simulink model "double_pendulum_model"  (R2020a)
settings: Solver=FixedStepAuto  StartTime=0.0  StopTime=5  FixedStep=1e-4  RelTol=1e-3  AbsTol=1e-3  EnableMultiTasking=on
undefined symbols (not defined in the file): sigbuilder_block, X, Y, Z
libraries: sm_lib x13, nesl_utility x8, simulink_extras x6, fl_lib x3
settings Model: Creator=Albert  LastModifiedBy=Albert
settings SolverCC: AutoScaleAbsTol=off
settings DataIOCC: LimitDataPoints=on  MaxDataPoints=10000
settings OptimizationCC: LifeSpan=inf
settings DebuggingCC: AllowSymbolicDim=off  SFUnexpectedBacktrackingDiag=warning  SFNoUnconditionalDefaultTransitionDiag=warning  SFExecutionAtInitializationDiag=none  ArithmeticOperatorsInVariantConditions=warning
settings SFSimCC: SimUseLocalCustomCode=off  CustomCodeUndefinedFunction=UseInterfaceOnly
settings RTWCC: RTWUseLocalCustomCode=off
settings CodeAppCC: StateflowObjectComments=on
settings GRTTargetCC: TargetLangStandard=C89/C90 (ANSI)
settings ConfigComp: CovMetricSettings=dw  CovSaveCumulativeToWorkspaceVar=on  CovSaveSingleToWorkspaceVar=on  CovExternalEMLEnable=off  CovSFcnEnable=off
settings SimscapeCC: SimscapeLogType=all  SimscapeLogSimulationStatistics=on  SimscapeLogDataHistory=10000

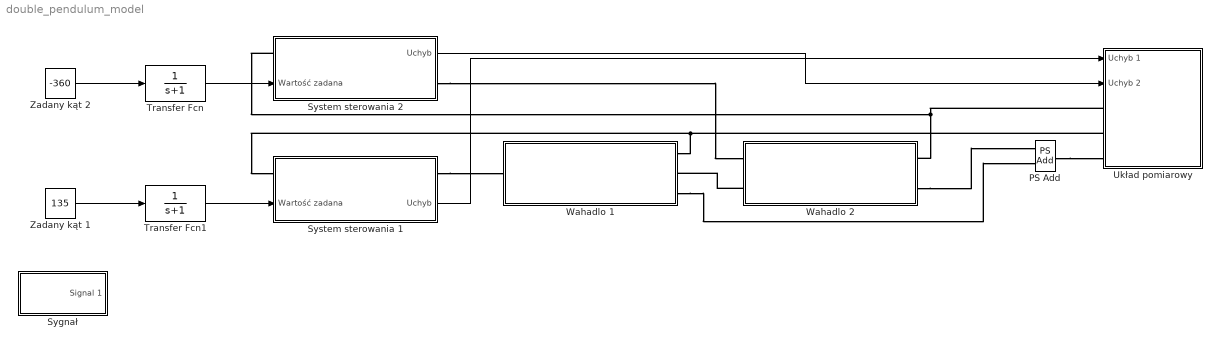
== system double_pendulum_model ==
  PS Add : fl_lib/Physical Signals/Functions/PS Add
  Sygnał : Subsystem  Tag=STV Subsys  LoadFcn=sigbuilder_block('load');  StartFcn=sigbuilder_block('start');  StopFcn=sigbuilder_block('stop');  ClipboardFcn=sigbuilder_block('clipboard');  mask(Sigbuilder block){tuvar=[0:10]}
      mask help: Simulink:masks:SigbuilderBlock_MD
      mask init:
      | if ~strcmp(get_param(bdroot(gcbh),'SimulationStatus'),'stopped') tuvar = sigbuilder_block('maskInit'); end
      settings: CopyFcn=sigbuilder_block('copy');  DeleteFcn=sigbuilder_block('delete');  ModelCloseFcn=sigbuilder_block('modelClose');  PreSaveFcn=sigbuilder_block('preSave');  PauseFcn=sigbuilder_block('pause');  ContinueFcn=sigbuilder_block('continue');  NameChangeFcn=sigbuilder_block('namechange');  OpenFcn=sigbuilder_block('open',[145.5 98.25 574.5 585.75 ]);  CloseFcn=sigbuilder_block('close');
      mask Display: plot(0, 0, 100, 100,[2, 2, 32, 32, 2], [68, 8, 8, 68, 68],[32, 2], [38, 38], [32, 19, 2],[53, 60, 44], [32, 17, 17, 2],[16, 16, 31, 31]);txt = getActiveGroup(gcbh);text(2, 100, txt,'verticalAlignment', 'top');
  System sterowania 1 : Subsystem
      settings: PortSchema="{\"entries\":[{\"content\":{\"sides\":[{\"content\":{\"connectorIds\":[\"LConn1\",\"In1\"]},\"type\":\"ConnectorPlacement.EquallySpacedRectSide\",\"uuid\":\"471d3fbd-ac29-446a-9427-316a60a908e6\"},{\"content\":{\"connectorIds\":[\"RConn1\",\"Out1\"],\"side\":\"RIGHT\"},\"type\":\"ConnectorPlacement.EquallySpacedRectSide\",\"uuid\":\"4c631136-7496-42ce-9ab5-63d38de6795d\"},{\"content\":{\"connectorIds\":[],\"side\":\"TOP\"},\"type\":\"ConnectorPlacement.EquallySpacedRectSide\",\"uuid\":\"d7f460c4-eb30-472b-8229-d5705620fcfc\"}]},\"type\":\"ConnectorPlacement.EquallySpacedConnector\",\"uuid\":\"0e46a79e-6a4e-432a-b324-1adcc0c34b7a\"}],\"packageUris\":[\"http://schema.mathworks.com/mf0/Connector/R2020b\"],\"version\":\"1.0\"}"
  System sterowania 2 : Subsystem
      settings: PortSchema="{\"entries\":[{\"content\":{\"sides\":[{\"content\":{\"connectorIds\":[\"LConn1\",\"In1\"]},\"type\":\"ConnectorPlacement.EquallySpacedRectSide\",\"uuid\":\"471d3fbd-ac29-446a-9427-316a60a908e6\"},{\"content\":{\"connectorIds\":[\"Out1\",\"RConn1\"],\"side\":\"RIGHT\"},\"type\":\"ConnectorPlacement.EquallySpacedRectSide\",\"uuid\":\"4c631136-7496-42ce-9ab5-63d38de6795d\"},{\"content\":{\"connectorIds\":[],\"side\":\"TOP\"},\"type\":\"ConnectorPlacement.EquallySpacedRectSide\",\"uuid\":\"d7f460c4-eb30-472b-8229-d5705620fcfc\"}]},\"type\":\"ConnectorPlacement.EquallySpacedConnector\",\"uuid\":\"0e46a79e-6a4e-432a-b324-1adcc0c34b7a\"}],\"packageUris\":[\"http://schema.mathworks.com/mf0/Connector/R2020b\"],\"version\":\"1.0\"}"
  Transfer Fcn : TransferFcn  Denominator=[1 1]
  Transfer Fcn1 : TransferFcn  Denominator=[1 1]
  Układ pomiarowy : Subsystem
  Wahadlo 1 : Subsystem
  Wahadlo 2 : Subsystem
  Zadany kąt 1 : Constant  Value=135
  Zadany kąt 2 : Constant  Value=-360
  wires:
  System sterowania 2/1(Uchyb) -> Układ pomiarowy/2(Uchyb 2)
  System sterowania 1/1(Uchyb) -> Układ pomiarowy/1(Uchyb 1)
  Zadany kąt 1/1 -> Transfer Fcn1/1
  Zadany kąt 2/1 -> Transfer Fcn/1
  Transfer Fcn/1 -> System sterowania 2/1(Wartość zadana)
  Transfer Fcn1/1 -> System sterowania 1/1(Wartość zadana)
  connections:
  Wahadlo 1/RConn1 -- System sterowania 1/LConn1 -- Układ pomiarowy/LConn2
  System sterowania 1/RConn1 -- Wahadlo 1/LConn1
  Wahadlo 2/LConn2 -- Wahadlo 1/RConn2
  System sterowania 2/LConn1 -- Układ pomiarowy/LConn1 -- Wahadlo 2/RConn1
  PS Add/RConn1 -- Układ pomiarowy/LConn3
  Wahadlo 1/RConn3 -- PS Add/LConn2
  Wahadlo 2/RConn2 -- PS Add/LConn1
  System sterowania 2/RConn1 -- Wahadlo 2/LConn1

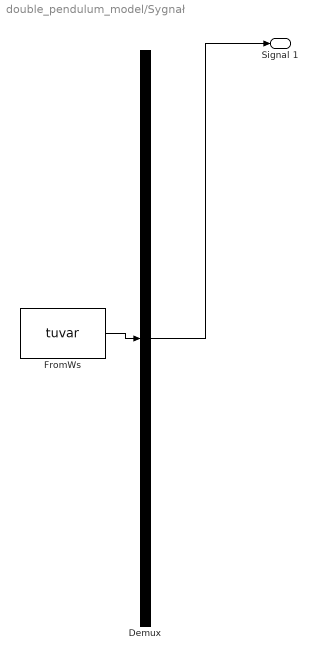
== system double_pendulum_model/Sygnał ==
  Demux : Demux  Tag=STV Demux  Outputs=1
      settings: DisplayOption=none
  FromWs : FromWorkspace  Tag=STV FromWs  VariableName=tuvar
      SigBuilderData=|
      | common.afterFinalStr = 'Extrapolate'
      | common.sampleTime = 0
      | dataSet.timeRange = [0 100]
      | dataSet.name = 'Group 1'
      | sbobj.Groups.Name = 'Group 1'
      | sbobj.Groups.Signals.Name = 'Signal 1'
      | sbobj.Groups.Signals.XData = [0 5 20 30 100]
      | sbobj.Groups.Signals.YData = [0 90 90 0 0]
      | sbobj.Groups.TimeRange = [0 100]
  Signal 1 : Outport  Tag=STV Outport  VectorParamsAs1DForOutWhenUnconnected=off
  wires:
  FromWs/1 -> Demux/1
  Demux/1 -> Signal 1/1

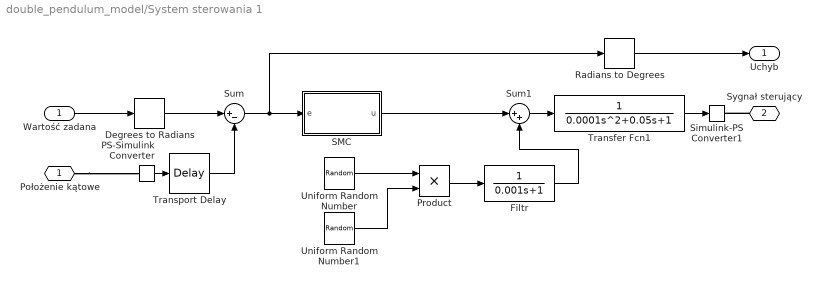
== system double_pendulum_model/System sterowania 1 ==
  Wartość zadana : Inport
  Degrees to Radians : simulink_extras/Transformations/Degrees to Radians
  Filtr : TransferFcn  Denominator=[0.001 1]
  PS-Simulink Converter : nesl_utility/PS-Simulink Converter  PhysicalDomain=network_engine_domain  SubClassName=ps_output  LeftPortType=input  RightPortType=output  PseudoPeriodic=off  Frequencies=[]  Unit=inherit  AffineConversion=off
      settings: SourceProductBaseCode=PW,SS
  Product : Product
  Radians to Degrees : simulink_extras/Transformations/Radians to Degrees
  SMC : Subsystem
  Simulink-PS Converter1 : nesl_utility/Simulink-PS Converter  PhysicalDomain=network_engine_domain  SubClassName=ps_input  LeftPortType=input  RightPortType=output  PseudoPeriodic=off  Frequencies=[]  NoiseDistribution=none  NoiseParameters=[]  Unit=1  AffineConversion=off  FilteringAndDerivatives=provide  SimscapeFilterOrder=1  InputFilterTimeConstant=0.001  UdotUserProvided=0
      settings: SourceProductBaseCode=PW,SS
  Sum : Sum  Inputs=|+-
  Sum1 : Sum  Inputs=|++
  Transfer Fcn1 : TransferFcn  Denominator=[0.0001 0.05 1]
  Transport Delay : TransportDelay  DelayTime=0.0001
  Uniform Random Number : UniformRandomNumber  Minimum=-0.05  Maximum=0.05
  Uniform Random Number1 : UniformRandomNumber  Minimum=-0.1  Maximum=0.1
  Położenie kątowe : PMIOPort  Side=Left
  Sygnał sterujący : PMIOPort  Port=2  Side=Right
  Uchyb : Outport
  wires:
  Degrees to Radians/1 -> Sum/1
  Wartość zadana/1 -> Degrees to Radians/1
  Sum/1 -> Radians to Degrees/1, SMC/1(e)
  PS-Simulink Converter/1 -> Transport Delay/1
  Transport Delay/1 -> Sum/2
  Uniform Random Number1/1 -> Product/2
  SMC/1(u) -> Sum1/1
  Uniform Random Number/1 -> Product/1
  Sum1/1 -> Transfer Fcn1/1
  Transfer Fcn1/1 -> Simulink-PS Converter1/1
  Product/1 -> Filtr/1
  Filtr/1 -> Sum1/2
  Radians to Degrees/1 -> Uchyb/1
  connections:
  Położenie kątowe/RConn1 -- PS-Simulink Converter/LConn1
  Sygnał sterujący/RConn1 -- Simulink-PS Converter1/RConn1

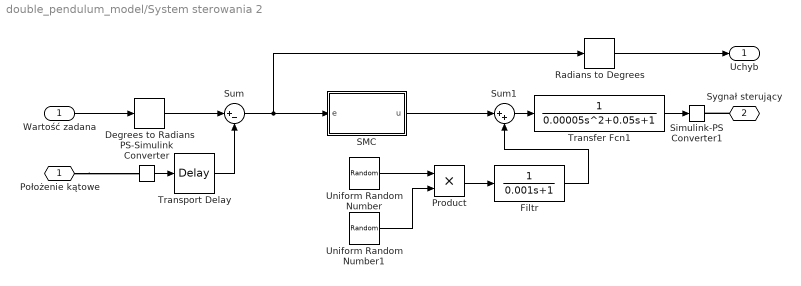
== system double_pendulum_model/System sterowania 2 ==
  Wartość zadana : Inport
  Degrees to Radians : simulink_extras/Transformations/Degrees to Radians
  Filtr : TransferFcn  Denominator=[0.001 1]
  PS-Simulink Converter : nesl_utility/PS-Simulink Converter  PhysicalDomain=network_engine_domain  SubClassName=ps_output  LeftPortType=input  RightPortType=output  PseudoPeriodic=off  Frequencies=[]  Unit=inherit  AffineConversion=off
      settings: SourceProductBaseCode=PW,SS
  Product : Product
  Radians to Degrees : simulink_extras/Transformations/Radians to Degrees
  SMC : Subsystem
  Simulink-PS Converter1 : nesl_utility/Simulink-PS Converter  PhysicalDomain=network_engine_domain  SubClassName=ps_input  LeftPortType=input  RightPortType=output  PseudoPeriodic=off  Frequencies=[]  NoiseDistribution=none  NoiseParameters=[]  Unit=1  AffineConversion=off  FilteringAndDerivatives=provide  SimscapeFilterOrder=1  InputFilterTimeConstant=0.001  UdotUserProvided=0
      settings: SourceProductBaseCode=PW,SS
  Sum : Sum  Inputs=|+-
  Sum1 : Sum  Inputs=|++
  Transfer Fcn1 : TransferFcn  Denominator=[0.00005 0.05 1]
  Transport Delay : TransportDelay  DelayTime=0.0001
  Uniform Random Number : UniformRandomNumber  Minimum=-0.05  Maximum=0.05
  Uniform Random Number1 : UniformRandomNumber  Minimum=-0.1  Maximum=0.1
  Położenie kątowe : PMIOPort  Side=Left
  Sygnał sterujący : PMIOPort  Port=2  Side=Right
  Uchyb : Outport
  wires:
  Sum/1 -> Radians to Degrees/1, SMC/1(e)
  Wartość zadana/1 -> Degrees to Radians/1
  Degrees to Radians/1 -> Sum/1
  PS-Simulink Converter/1 -> Transport Delay/1
  Transport Delay/1 -> Sum/2
  SMC/1(u) -> Sum1/1
  Uniform Random Number/1 -> Product/1
  Uniform Random Number1/1 -> Product/2
  Transfer Fcn1/1 -> Simulink-PS Converter1/1
  Sum1/1 -> Transfer Fcn1/1
  Product/1 -> Filtr/1
  Filtr/1 -> Sum1/2
  Radians to Degrees/1 -> Uchyb/1
  connections:
  Położenie kątowe/RConn1 -- PS-Simulink Converter/LConn1
  Sygnał sterujący/RConn1 -- Simulink-PS Converter1/RConn1

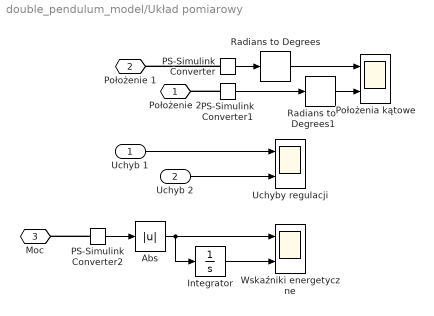
== system double_pendulum_model/Układ pomiarowy ==
  Uchyb 1 : Inport
  Uchyb 2 : Inport  Port=2
  Abs : Abs
  Integrator : Integrator
  PS-Simulink Converter : nesl_utility/PS-Simulink Converter  PhysicalDomain=network_engine_domain  SubClassName=ps_output  LeftPortType=input  RightPortType=output  PseudoPeriodic=off  Frequencies=[]  Unit=inherit  AffineConversion=off
      settings: SourceProductBaseCode=PW,SS
  PS-Simulink Converter1 : nesl_utility/PS-Simulink Converter  PhysicalDomain=network_engine_domain  SubClassName=ps_output  LeftPortType=input  RightPortType=output  PseudoPeriodic=off  Frequencies=[]  Unit=inherit  AffineConversion=off
      settings: SourceProductBaseCode=PW,SS
  PS-Simulink Converter2 : nesl_utility/PS-Simulink Converter  PhysicalDomain=network_engine_domain  SubClassName=ps_output  LeftPortType=input  RightPortType=output  PseudoPeriodic=off  Frequencies=[]  Unit=inherit  AffineConversion=off
      settings: SourceProductBaseCode=PW,SS
  Położenia kątowe : Scope  NumInputPorts=2
  Radians to Degrees : simulink_extras/Transformations/Radians to Degrees
  Radians to Degrees1 : simulink_extras/Transformations/Radians to Degrees
  Uchyby regulacji : Scope  NumInputPorts=2
  Wskaźniki energetyczne : Scope  NumInputPorts=2
  Położenie 2 : PMIOPort  Side=Left
  Położenie 1 : PMIOPort  Port=2  Side=Left
  Moc : PMIOPort  Port=3  Side=Left
  wires:
  Uchyb 2/1 -> Uchyby regulacji/2
  Uchyb 1/1 -> Uchyby regulacji/1
  Integrator/1 -> Wskaźniki energetyczne/2
  PS-Simulink Converter/1 -> Radians to Degrees/1
  Radians to Degrees/1 -> Położenia kątowe/1
  Radians to Degrees1/1 -> Położenia kątowe/2
  PS-Simulink Converter1/1 -> Radians to Degrees1/1
  PS-Simulink Converter2/1 -> Abs/1
  Abs/1 -> Wskaźniki energetyczne/1, Integrator/1
  connections:
  PS-Simulink Converter1/LConn1 -- Położenie 2/RConn1
  PS-Simulink Converter/LConn1 -- Położenie 1/RConn1
  PS-Simulink Converter2/LConn1 -- Moc/RConn1

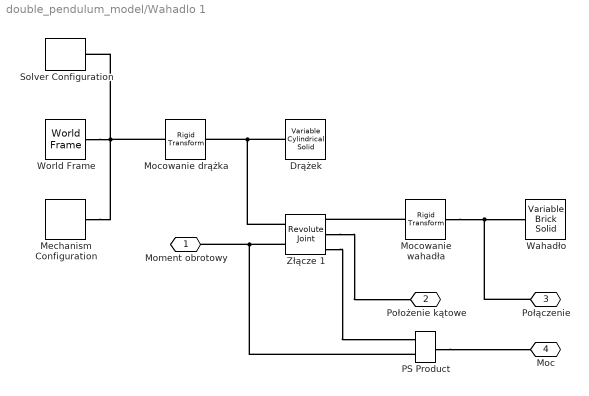
== system double_pendulum_model/Wahadlo 1 ==
  Drążek : sm_lib/Body Elements/Variable Mass/Variable Cylindrical Solid  LengthType=Constant  Length=50  LengthUnits=cm  RadiusType=Constant  Radius=30  RadiusUnits=mm  MassType=CalculateFromGeometry  InitialMassType=Specified  InitialMass=1  InitialMassUnits=kg  Density=1000  DensityUnits=kg/m^3  SenseRadius=off  SenseLength=off  SenseMass=off  SenseCenterOfMass=off  SenseInertiaMatrix=off  GraphicType=FromGeometry  MarkerShape=Sphere  MarkerSize=10  GraphicVisPropType=SimpleVisualProperties  GraphicDiffuseColor=[1.0 1.0 1.0]  GraphicSpecularColor=[0.5 0.5 0.5 1.0]  GraphicAmbientColor=[0.15 0.15 0.15 1.0]  GraphicEmissiveColor=[0.0 0.0 0.0 1.0]  GraphicShininess=75  GraphicOpacity=1.0
      settings: SourceProductBaseCode=MS
  Mechanism Configuration : sm_lib/Utilities/Mechanism Configuration  UniformGravity=Constant  GravityVector=[0 0 -9.80665]  GravityVectorUnits=m/s^2  GravityUnits=m/s^2  LinearizationDelta=0.001  JointModeTransitionNonlinearIterations=2
  Mocowanie drążka : sm_lib/Frames and Transforms/Rigid Transform  TranslationMethod=None  TranslationStandardOffset=0  TranslationLengthUnit=m  TranslationStandardAxis=+Z  TranslationCartesianOffset=[0 0 0]  TranslationROffset=0  TranslationROffsetUnits=m  TranslationZOffset=0  TranslationZOffsetUnits=m  TranslationThetaOffset=0  TranslationThetaOffsetUnits=deg  RotationMethod=RotationSequence  RotationAngleUnits=deg  RotationStandardAxis=+Z  RotationAngle=0.0  RotationArbitraryAxis=[0 0 1]  FollAlignAxisA=+X  BaseAlignAxisA=+Y  FollAlignAxisB=+Y  BaseAlignAxisB=+Z  RotationSequenceAxes=FollowerAxes  RotationSequence=YXY  RotationSequenceAngles=[0 90 0]  RotationSequenceAnglesUnits=deg  RotationMatrix=[1 0 0; 0 1 0; 0 0 1]
  Mocowanie wahadła : sm_lib/Frames and Transforms/Rigid Transform  TranslationMethod=Cartesian  TranslationStandardOffset=0  TranslationLengthUnit=cm  TranslationStandardAxis=+Z  TranslationCartesianOffset=[0 -14 25]  TranslationROffset=0  TranslationROffsetUnits=m  TranslationZOffset=0  TranslationZOffsetUnits=m  TranslationThetaOffset=0  TranslationThetaOffsetUnits=deg  RotationMethod=RotationSequence  RotationAngleUnits=deg  RotationStandardAxis=+Z  RotationAngle=0.0  RotationArbitraryAxis=[0 0 1]  FollAlignAxisA=+X  BaseAlignAxisA=+Y  FollAlignAxisB=+Y  BaseAlignAxisB=+Z  RotationSequenceAxes=FollowerAxes  RotationSequence=XYZ  RotationSequenceAngles=[0 0 90]  RotationSequenceAnglesUnits=deg  RotationMatrix=[1 0 0; 0 1 0; 0 0 1]
  PS Product : fl_lib/Physical Signals/Functions/PS Product
  Solver Configuration : nesl_utility/Solver Configuration  PhysicalDomain=network_engine_domain  SubClassName=solver  LeftPortType=input  RightPortType=generic  Tones=[]  Harmonics=[]  SimulateNoise=off  Profile=off  UseLocalSampling=off  EnableSwitchedLinearOptims=on  FrequencyDomain=off  UseCCode=off  RelTol=0.001  AbsTol=1e-06  MinStep=1e-09  ToWorkspace=off  RevertToSquareIcSolve=off  NumHomotopyIterations=100  PhasorMode=off  PhasorModeNumHarmonics=1  DoDC=off  ResidualTolerance=1e-09  UseLocalSolver=off  LocalSolverChoice=NE_BACKWARD_EULER_ADVANCER  LocalSolverSampleTime=0.001  DoFixedCost=off  MaxNonlinIter=3  MaxModeIter=2  ComputeImpulses=off  ImpulseIterations=2  LinearAlgebra=Sparse  EquationFormulation=NE_TIME_EF  DelaysMemoryBudget=1024  AutomaticFiltering=on  FilteringTimeConstant=0.001  PartitionStorageMethod=AS_NEEDED  PartitionMemoryBudget=1024  PartitionMethod=FAST
      settings: SourceProductBaseCode=PW,SS
  Wahadło : sm_lib/Body Elements/Variable Mass/Variable Brick Solid  XLengthType=Constant  XLength=30  XLengthUnits=cm  YLengthType=Constant  YLength=5  YLengthUnits=cm  ZLengthType=Constant  ZLength=20  ZLengthUnits=mm  MassType=CalculateFromGeometry  InitialMassType=Specified  InitialMass=1  InitialMassUnits=kg  Density=5000  DensityUnits=kg/m^3  SenseXLength=off  SenseYLength=off  SenseZLength=off  SenseMass=off  SenseCenterOfMass=off  SenseInertiaMatrix=off  GraphicType=FromGeometry  MarkerShape=Sphere  MarkerSize=10  GraphicVisPropType=SimpleVisualProperties  GraphicDiffuseColor=[1.0 0.0 0.0]  GraphicSpecularColor=[0.5 0.5 0.5 1.0]  GraphicAmbientColor=[0.15 0.15 0.15 1.0]  GraphicEmissiveColor=[0.0 0.0 0.0 1.0]  GraphicShininess=75  GraphicOpacity=0.5
      settings: SourceProductBaseCode=MS
  World Frame : sm_lib/Frames and Transforms/World Frame
  Złącze 1 : sm_lib/Joints/Revolute Joint  JointMode=Normal  SenseConstraintForce=off  SenseConstraintForceX=off  SenseConstraintForceY=off  SenseConstraintForceZ=off  SenseConstraintTorque=off  SenseConstraintTorqueX=off  SenseConstraintTorqueY=off  SenseConstraintTorqueZ=off  SenseTotalForce=off  SenseTotalForceX=off  SenseTotalForceY=off  SenseTotalForceZ=off  SenseTotalTorque=off  SenseTotalTorqueX=off  SenseTotalTorqueY=off  SenseTotalTorqueZ=off  CompositeWrenchDir=FollowerOnBase  CompositeWrenchFrame=BaseFrame  EquilibriumPosition=0  EquilibriumPositionUnits=deg  SpringStiffness=0  SpringStiffnessUnits=N*m/deg  DampingCoefficient=0.001  DampingCoefficientUnits=N*m/(deg/s)  TorqueActuationMode=InputTorque  MotionActuationMode=ComputedMotion  SensePosition=on  SenseVelocity=on  SenseAcceleration=off  SenseTorqueForce=off  SenseLowerLimitTorqueForce=off  SenseUpperLimitTorqueForce=off  LowerLimitSpecify=off  LowerLimitBound=-90  LowerLimitBoundUnits=deg  LowerLimitStiffness=1e4  LowerLimitStiffnessUnits=N*m/deg  LowerLimitDamping=10  LowerLimitDampingUnits=N*m/(deg/s)  LowerLimitTransitionRegionWidth=0.1  LowerLimitTransitionRegionWidthUnits=deg  UpperLimitSpecify=off  UpperLimitBound=90  UpperLimitBoundUnits=deg  UpperLimitStiffness=1e4  UpperLimitStiffnessUnits=N*m/deg  UpperLimitDamping=10  UpperLimitDampingUnits=N*m/(deg/s)  UpperLimitTransitionRegionWidth=0.1  UpperLimitTransitionRegionWidthUnits=deg  PositionTargetSpecify=off  PositionTargetPriority=High  PositionTargetValue=0  PositionTargetValueUnits=deg  VelocityTargetSpecify=off  VelocityTargetPriority=High  VelocityTargetValue=0  VelocityTargetValueUnits=deg/s
  Moment obrotowy : PMIOPort  Side=Left
  Położenie kątowe : PMIOPort  Port=2  Side=Right
  Połączenie : PMIOPort  Port=3  Side=Right
  Moc : PMIOPort  Port=4  Side=Right
  connections:
  Złącze 1/RConn2 -- Położenie kątowe/RConn1
  World Frame/RConn1 -- Mechanism Configuration/RConn1 -- Mocowanie drążka/LConn1 -- Solver Configuration/RConn1
  Złącze 1/LConn2 -- PS Product/LConn2 -- Moment obrotowy/RConn1
  Drążek/RConn1 -- Złącze 1/LConn1 -- Mocowanie drążka/RConn1
  Mocowanie wahadła/RConn1 -- Połączenie/RConn1 -- Wahadło/RConn1
  Mocowanie wahadła/LConn1 -- Złącze 1/RConn1
  PS Product/RConn1 -- Moc/RConn1
  Złącze 1/RConn3 -- PS Product/LConn1

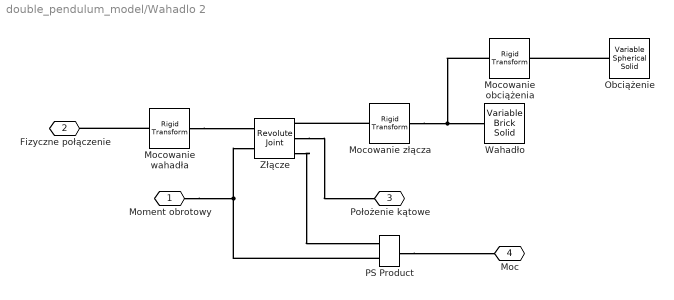
== system double_pendulum_model/Wahadlo 2 ==
  Mocowanie obciążenia : sm_lib/Frames and Transforms/Rigid Transform  TranslationMethod=Cartesian  TranslationStandardOffset=0  TranslationLengthUnit=cm  TranslationStandardAxis=+Z  TranslationCartesianOffset=[-10 0 1]  TranslationROffset=0  TranslationROffsetUnits=m  TranslationZOffset=0  TranslationZOffsetUnits=m  TranslationThetaOffset=0  TranslationThetaOffsetUnits=deg  RotationMethod=None  RotationAngleUnits=deg  RotationStandardAxis=+Z  RotationAngle=0.0  RotationArbitraryAxis=[0 0 1]  FollAlignAxisA=+X  BaseAlignAxisA=+Y  FollAlignAxisB=+Y  BaseAlignAxisB=+Z  RotationSequenceAxes=FollowerAxes  RotationSequence=XYZ  RotationSequenceAngles=[0 0 0]  RotationSequenceAnglesUnits=deg  RotationMatrix=[1 0 0; 0 1 0; 0 0 1]
  Mocowanie wahadła : sm_lib/Frames and Transforms/Rigid Transform  TranslationMethod=Cartesian  TranslationStandardOffset=0  TranslationLengthUnit=cm  TranslationStandardAxis=+Z  TranslationCartesianOffset=[-10 0 2]  TranslationROffset=0  TranslationROffsetUnits=m  TranslationZOffset=0  TranslationZOffsetUnits=m  TranslationThetaOffset=0  TranslationThetaOffsetUnits=deg  RotationMethod=None  RotationAngleUnits=deg  RotationStandardAxis=+Z  RotationAngle=0.0  RotationArbitraryAxis=[0 0 1]  FollAlignAxisA=+X  BaseAlignAxisA=+Y  FollAlignAxisB=+Y  BaseAlignAxisB=+Z  RotationSequenceAxes=FollowerAxes  RotationSequence=XYZ  RotationSequenceAngles=[0 0 0]  RotationSequenceAnglesUnits=deg  RotationMatrix=[1 0 0; 0 1 0; 0 0 1]
  Mocowanie złącza : sm_lib/Frames and Transforms/Rigid Transform  TranslationMethod=Cartesian  TranslationStandardOffset=0  TranslationLengthUnit=cm  TranslationStandardAxis=+Z  TranslationCartesianOffset=[-10 0 0]  TranslationROffset=0  TranslationROffsetUnits=m  TranslationZOffset=0  TranslationZOffsetUnits=m  TranslationThetaOffset=0  TranslationThetaOffsetUnits=deg  RotationMethod=None  RotationAngleUnits=deg  RotationStandardAxis=+Z  RotationAngle=0.0  RotationArbitraryAxis=[0 0 1]  FollAlignAxisA=+X  BaseAlignAxisA=+Y  FollAlignAxisB=+Y  BaseAlignAxisB=+Z  RotationSequenceAxes=FollowerAxes  RotationSequence=XYZ  RotationSequenceAngles=[0 0 0]  RotationSequenceAnglesUnits=deg  RotationMatrix=[1 0 0; 0 1 0; 0 0 1]
  Obciążenie : sm_lib/Body Elements/Variable Mass/Variable Spherical Solid  RadiusType=Constant  Radius=50  RadiusUnits=mm  MassType=CalculateFromGeometry  InitialMassType=Specified  InitialMass=1  InitialMassUnits=kg  Density=500  DensityUnits=kg/m^3  SenseRadius=off  SenseMass=off  SenseCenterOfMass=off  SenseInertiaMatrix=off  GraphicType=FromGeometry  MarkerShape=Sphere  MarkerSize=10  GraphicVisPropType=SimpleVisualProperties  GraphicDiffuseColor=[1.0 0.6 0.2]  GraphicSpecularColor=[0.5 0.5 0.5 1.0]  GraphicAmbientColor=[0.15 0.15 0.15 1.0]  GraphicEmissiveColor=[0.0 0.0 0.0 1.0]  GraphicShininess=75  GraphicOpacity=0.8
      settings: SourceProductBaseCode=MS
  PS Product : fl_lib/Physical Signals/Functions/PS Product
  Wahadło : sm_lib/Body Elements/Variable Mass/Variable Brick Solid  XLengthType=Constant  XLength=20  XLengthUnits=cm  YLengthType=Constant  YLength=5  YLengthUnits=cm  ZLengthType=Constant  ZLength=20  ZLengthUnits=mm  MassType=CalculateFromGeometry  InitialMassType=Specified  InitialMass=1  InitialMassUnits=kg  Density=3000  DensityUnits=kg/m^3  SenseXLength=off  SenseYLength=off  SenseZLength=off  SenseMass=off  SenseCenterOfMass=off  SenseInertiaMatrix=off  GraphicType=FromGeometry  MarkerShape=Sphere  MarkerSize=10  GraphicVisPropType=SimpleVisualProperties  GraphicDiffuseColor=[0.8 0.0 0.4]  GraphicSpecularColor=[0.5 0.5 0.5 1.0]  GraphicAmbientColor=[0.15 0.15 0.15 1.0]  GraphicEmissiveColor=[0.0 0.0 0.0 1.0]  GraphicShininess=75  GraphicOpacity=0.5
      settings: SourceProductBaseCode=MS
  Złącze : sm_lib/Joints/Revolute Joint  JointMode=Normal  SenseConstraintForce=off  SenseConstraintForceX=off  SenseConstraintForceY=off  SenseConstraintForceZ=off  SenseConstraintTorque=off  SenseConstraintTorqueX=off  SenseConstraintTorqueY=off  SenseConstraintTorqueZ=off  SenseTotalForce=off  SenseTotalForceX=off  SenseTotalForceY=off  SenseTotalForceZ=off  SenseTotalTorque=off  SenseTotalTorqueX=off  SenseTotalTorqueY=off  SenseTotalTorqueZ=off  CompositeWrenchDir=FollowerOnBase  CompositeWrenchFrame=BaseFrame  EquilibriumPosition=0  EquilibriumPositionUnits=deg  SpringStiffness=0  SpringStiffnessUnits=N*m/deg  DampingCoefficient=0.001  DampingCoefficientUnits=N*m/(deg/s)  TorqueActuationMode=InputTorque  MotionActuationMode=ComputedMotion  SensePosition=on  SenseVelocity=on  SenseAcceleration=off  SenseTorqueForce=off  SenseLowerLimitTorqueForce=off  SenseUpperLimitTorqueForce=off  LowerLimitSpecify=off  LowerLimitBound=-90  LowerLimitBoundUnits=deg  LowerLimitStiffness=1e4  LowerLimitStiffnessUnits=N*m/deg  LowerLimitDamping=10  LowerLimitDampingUnits=N*m/(deg/s)  LowerLimitTransitionRegionWidth=0.1  LowerLimitTransitionRegionWidthUnits=deg  UpperLimitSpecify=off  UpperLimitBound=90  UpperLimitBoundUnits=deg  UpperLimitStiffness=1e4  UpperLimitStiffnessUnits=N*m/deg  UpperLimitDamping=10  UpperLimitDampingUnits=N*m/(deg/s)  UpperLimitTransitionRegionWidth=0.1  UpperLimitTransitionRegionWidthUnits=deg  PositionTargetSpecify=off  PositionTargetPriority=High  PositionTargetValue=0  PositionTargetValueUnits=deg  VelocityTargetSpecify=off  VelocityTargetPriority=High  VelocityTargetValue=0  VelocityTargetValueUnits=deg/s
  Moment obrotowy : PMIOPort  Side=Left
  Fizyczne połączenie : PMIOPort  Port=2  Side=Left
  Położenie kątowe : PMIOPort  Port=3  Side=Right
  Moc : PMIOPort  Port=4  Side=Right
  connections:
  Mocowanie złącza/LConn1 -- Złącze/RConn1
  Złącze/RConn2 -- Położenie kątowe/RConn1
  Mocowanie złącza/RConn1 -- Wahadło/RConn1 -- Mocowanie obciążenia/LConn1
  Mocowanie wahadła/RConn1 -- Złącze/LConn1
  Mocowanie wahadła/LConn1 -- Fizyczne połączenie/RConn1
  Moment obrotowy/RConn1 -- PS Product/LConn2 -- Złącze/LConn2
  Obciążenie/RConn1 -- Mocowanie obciążenia/RConn1
  Złącze/RConn3 -- PS Product/LConn1
  PS Product/RConn1 -- Moc/RConn1

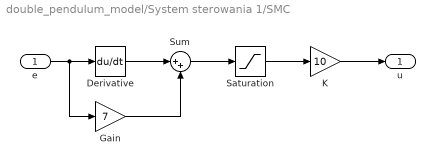
== system double_pendulum_model/System sterowania 1/SMC ==
  e : Inport
  Derivative : Derivative
  Gain : Gain  Gain=7
  K : Gain  Gain=10
  Saturation : Saturate  UpperLimit=1  LowerLimit=-1
  Sum : Sum  Inputs=|++
  u : Outport
  wires:
  e/1 -> Gain/1, Derivative/1
  Derivative/1 -> Sum/1
  Gain/1 -> Sum/2
  Sum/1 -> Saturation/1
  Saturation/1 -> K/1
  K/1 -> u/1

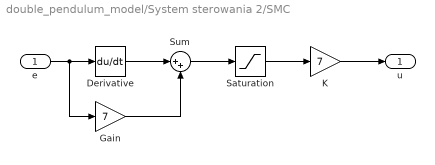
== system double_pendulum_model/System sterowania 2/SMC ==
  e : Inport
  Derivative : Derivative
  Gain : Gain  Gain=7
  K : Gain  Gain=7
  Saturation : Saturate  UpperLimit=1  LowerLimit=-1
  Sum : Sum  Inputs=|++
  u : Outport
  wires:
  e/1 -> Gain/1, Derivative/1
  Derivative/1 -> Sum/1
  Gain/1 -> Sum/2
  Sum/1 -> Saturation/1
  Saturation/1 -> K/1
  K/1 -> u/1
